simulink model "OverallStateflow"  (R2021a)
settings: Solver=FixedStepDiscrete  StartTime=0.0  StopTime=10.0  FixedStep=0.1  RelTol=1e-3  EnableMultiTasking=on
settings Model: Creator=kylec  LastModifiedBy=johna
settings SolverCC: AlgebraicLoopSolver=TrustRegion  AutoInsertRateTranBlk=on
settings DataIOCC: LimitDataPoints=on
settings OptimizationCC: LifeSpan=inf
settings DebuggingCC: AllowSymbolicDim=off  SFUnexpectedBacktrackingDiag=warning  SFNoUnconditionalDefaultTransitionDiag=warning  SFExecutionAtInitializationDiag=none  ArithmeticOperatorsInVariantConditions=warning
settings SFSimCC: SimUseLocalCustomCode=off  CustomCodeUndefinedFunction=UseInterfaceOnly
settings RTWCC: RTWUseLocalCustomCode=off
settings CodeAppCC: StateflowObjectComments=on
settings GRTTargetCC: TargetLangStandard=C89/C90 (ANSI)
settings ConfigComp: CovMetricSettings=dw  CovSaveCumulativeToWorkspaceVar=on  CovSaveSingleToWorkspaceVar=on  CovExternalEMLEnable=off  CovSFcnEnable=off

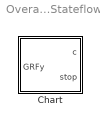
== system OverallStateflow ==
  Chart : Stateflow chart  TreatAsAtomicUnit=on

== stateflow chart OverallStateflow/Chart ==
  state Init
    entry:
    c = 2;
  state Command
    entry:
    c = 3;
    state Stand
    state Stance
    state Flight
    state Sit
    (default) -> Stand
    Stand -> Stance
    Flight -> Stance : [GRFy > 0]
    Stance -> Flight [order 2] : [GRFy == 0]
    Stance -> Sit [order 1]
  state Danger
  state Deinitiate
    entry:
    c = 4;
  (default) -> Init
  Init -> Command : after(3, sec)
  Command -> Danger [order 2]
  Command -> Deinitiate [order 1]
  Deinitiate -> (junction 36) : after(3,sec)
  (junction 36) -> Deinitiate : {stop = 1}
  data: GRFy input; c output; stop output =0
